simulink model "zad5"  (R2022b)
settings: Solver=VariableStepAuto  StartTime=0.0  StopTime=13  RelTol=1e-3
libraries: simulink_extras x5, simulink x4, hdlsllib x1
settings Model: Creator=user  LastModifiedBy=Karolina
settings SolverCC: AlgebraicLoopSolver=TrustRegion
settings DebuggingCC: UnconnectedInputMsg=warning  UnconnectedOutputMsg=warning  UnconnectedLineMsg=warning  SFMachineParentedDataDiag=warning
settings ModelReferenceCC: EnableRefExpFcnMdlSchedulingChecks=on
settings SFSimCC: CustomCodeUndefinedFunction=UseInterfaceOnly

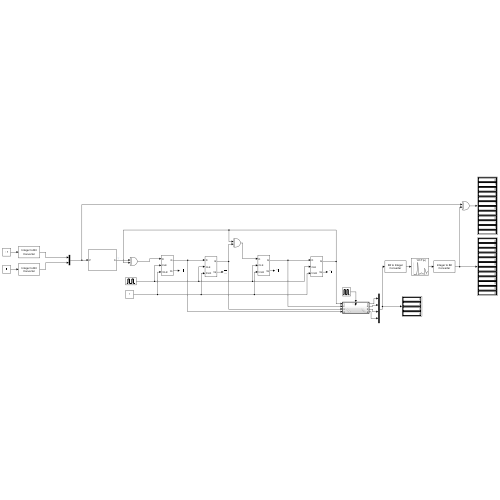
[thumbnail: Simulink's stored preview of the top-level diagram]
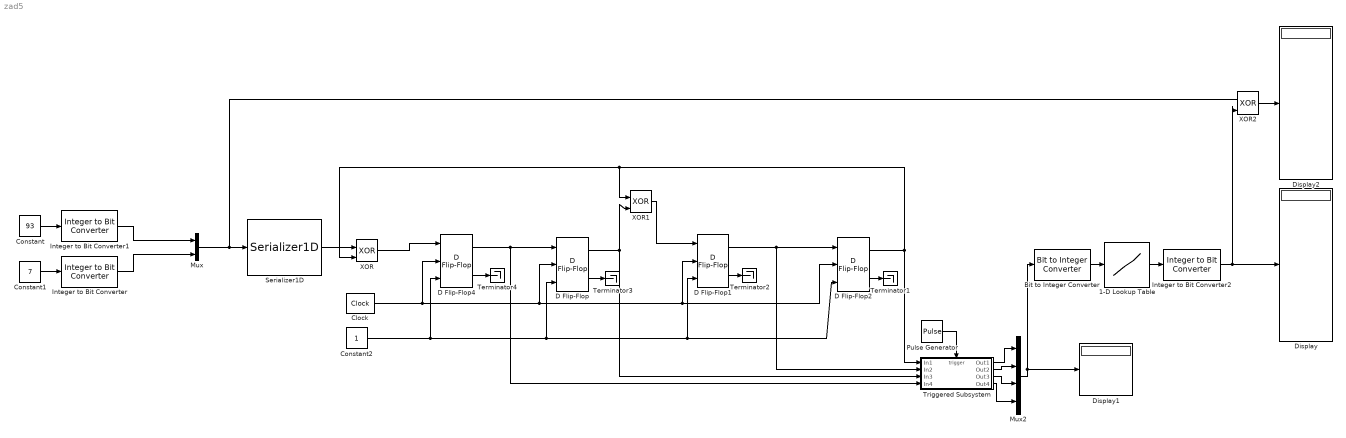
== system zad5 ==
  1-D Lookup Table : Lookup_n-D  NumberOfTableDimensions=1  BreakpointsForDimension1=[0;1;2;4;5;7;8;10;13;18;19;22;24]  Table=[0;1;2;4;32;2048;8;64;256;16;1024;128;512]  ExtrapMethod=Clip  InternalRulePriority=Speed  OutDataTypeStr=uint16  RndMeth=Simplest
  Bit to Integer Converter : simulink/Logic and Bit Operations/Bit to Integer Converter  nbits=4  bitOrder=MSB first  signedOutputValues=Unsigned  outDtype=Inherit via internal rule  outDtypeSigned=Inherit via internal rule
  Clock : simulink_extras/Flip Flops/Clock  period=1
  Constant : Constant  Value=93
  Constant1 : Constant  Value=7
  Constant2 : Constant
  D Flip-Flop{,1..2,4} (4 alike) : simulink_extras/Flip Flops/D Flip-Flop
  Display : Display
      settings: Decimation=4
  Display1 : Display
      settings: Decimation=4
  Display2 : Display
      settings: Decimation=4
  Integer to Bit Converter : simulink/Logic and Bit Operations/Integer to Bit Converter  nbits=4  signedInputValues=Unsigned  bitOrder=MSB first  outDtype=boolean
      settings: LibrarySourceBlock=|
      | commutil2/Integer to Bit
      | Converter
  Integer to Bit Converter1 : simulink/Logic and Bit Operations/Integer to Bit Converter  nbits=8  signedInputValues=Unsigned  bitOrder=MSB first  outDtype=boolean
      settings: LibrarySourceBlock=|
      | commutil2/Integer to Bit
      | Converter
  Integer to Bit Converter2 : simulink/Logic and Bit Operations/Integer to Bit Converter  nbits=12  signedInputValues=Unsigned  bitOrder=MSB first  outDtype=Inherit via internal rule
  Mux : Mux  Inputs=2
  Mux2 : Mux
  Pulse Generator : DiscretePulseGenerator  PulseType=Time based  Period=1  PulseWidth=5  PhaseDelay=12.5
  Serializer1D : hdlsllib/HDL Operations/Serializer1D  Ratio=12  IdleCycles=0  validIn=off  startOut=off  validOut=off  inputDataDimensions=-1  inputSampleTime=12  inputSignalType=auto
  Terminator{1..4} (4 alike) : Terminator
  Triggered Subsystem : Subsystem  TreatAsAtomicUnit=on
  XOR : Logic  Operator=XOR  IconShape=distinctive  AllPortsSameDT=off  OutDataTypeStr=boolean
  XOR1 : Logic  Operator=XOR  IconShape=distinctive  AllPortsSameDT=off  OutDataTypeStr=boolean
  XOR2 : Logic  Operator=XOR  IconShape=distinctive  AllPortsSameDT=off  OutDataTypeStr=boolean
  wires:
  Constant/1 -> Integer to Bit Converter1/1
  Constant1/1 -> Integer to Bit Converter/1
  Serializer1D/1 -> XOR/1
  D Flip-Flop2/1 -> Triggered Subsystem/1(In1), XOR/2, XOR1/1
  Constant2/1 -> D Flip-Flop4/3, D Flip-Flop/3, D Flip-Flop1/3, D Flip-Flop2/3
  Clock/1 -> D Flip-Flop4/2, D Flip-Flop/2, D Flip-Flop2/2, D Flip-Flop1/2
  Pulse Generator/1 -> Triggered Subsystem/Trigger
  D Flip-Flop2/2 -> Terminator1/1
  D Flip-Flop1/2 -> Terminator2/1
  D Flip-Flop/2 -> Terminator3/1
  Integer to Bit Converter1/1 -> Mux/1
  Triggered Subsystem/4(Out4) -> Mux2/4
  Triggered Subsystem/3(Out3) -> Mux2/3
  Triggered Subsystem/2(Out2) -> Mux2/2
  Triggered Subsystem/1(Out1) -> Mux2/1
  Mux2/1 -> Display1/1, Bit to Integer Converter/1
  Integer to Bit Converter/1 -> Mux/2
  Bit to Integer Converter/1 -> 1-D Lookup Table/1
  1-D Lookup Table/1 -> Integer to Bit Converter2/1
  Integer to Bit Converter2/1 -> XOR2/2, Display/1
  XOR2/1 -> Display2/1
  D Flip-Flop4/1 -> Triggered Subsystem/4(In4), D Flip-Flop/1
  D Flip-Flop4/2 -> Terminator4/1
  XOR/1 -> D Flip-Flop4/1
  D Flip-Flop1/1 -> Triggered Subsystem/2(In2), D Flip-Flop2/1
  XOR1/1 -> D Flip-Flop1/1
  D Flip-Flop/1 -> Triggered Subsystem/3(In3), XOR1/2
  Mux/1 -> XOR2/1, Serializer1D/1

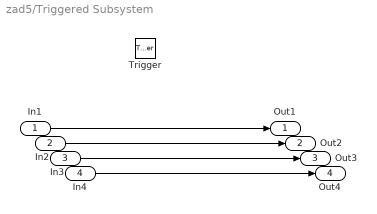
== system zad5/Triggered Subsystem ==
  In1 : Inport
  In2 : Inport  Port=2
  In3 : Inport  Port=3
  In4 : Inport  Port=4
  Trigger : TriggerPort  VariantControl=Variant
  Out1 : Outport  VectorParamsAs1DForOutWhenUnconnected=off
  Out2 : Outport  Port=2  VectorParamsAs1DForOutWhenUnconnected=off
  Out3 : Outport  Port=3  VectorParamsAs1DForOutWhenUnconnected=off
  Out4 : Outport  Port=4  VectorParamsAs1DForOutWhenUnconnected=off
  wires:
  In1/1 -> Out1/1
  In2/1 -> Out2/1
  In3/1 -> Out3/1
  In4/1 -> Out4/1
